simulink subsystem "Vehicle_Controller_SM_v4"  (R2023b)
settings: Solver=VariableStepAuto  StartTime=0.0  StopTime=10.0  RelTol=1e-3
undefined symbols (not defined in the file): chassis, powertrain, sensor, sim, suspension, tvs
libraries: lib_newData_range_check x4, dspstat3 x1, simulink x1
settings Model: Creator=Inver  LastModifiedBy=bowen
settings OptimizationCC: ReuseModelBlockBuffer=off

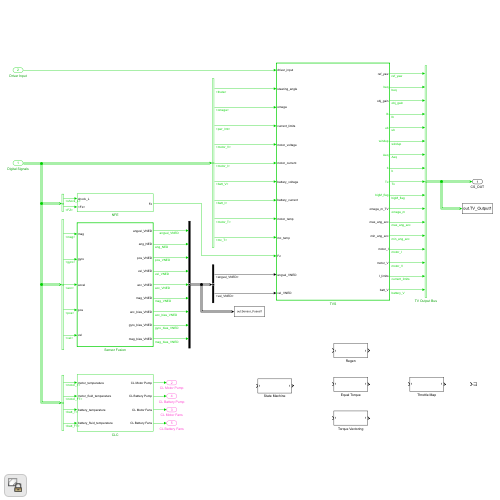
[thumbnail: Simulink's stored preview of the top-level diagram]
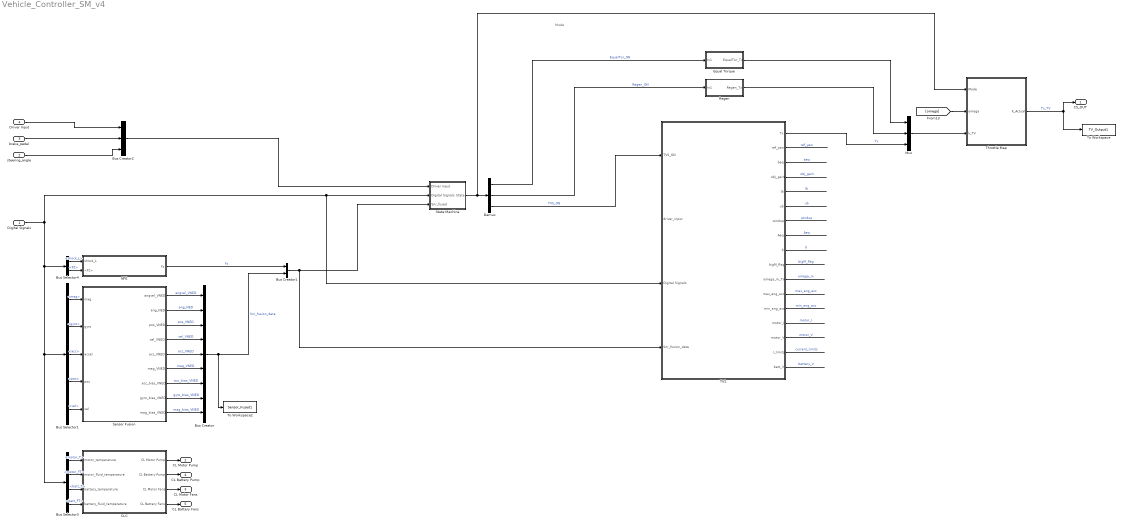
== system Vehicle_Controller_SM_v4 ==
  note: Mode
  Digital Signals : Inport
  steering_angle : Inport  Port=2
  brake_pedal : Inport  Port=3
  Driver Input : Inport  Port=4
  Bus Creator : BusCreator  Inputs=9
  Bus Creator1 : BusCreator  Inputs=2
  Bus Creator2 : BusCreator  Inputs=3
  Bus Selector1 : BusSelector  OutputSignals=Navigation Sensors.mag,Navigation Sensors.gyro,Navigation Sensors.acc,Navigation Sensors.pos,Navigation Sensors.vel
  Bus Selector3 : BusSelector  OutputSignals=Cooling Sensors.motor_T,Cooling Sensors.motor_FT,Cooling Sensors.batt_T,Cooling Sensors.batt_FT
  Bus Selector4 : BusSelector  OutputSignals=Corner Dynamics Sensors.shock_L,Corner Dynamics Sensors.FZ
  CLC : Subsystem
  Demux : Demux  Outputs=3
  Equal Torque : Subsystem
  Mux : Mux  Inputs=3
  NFE : Subsystem
  Regen : Subsystem
  Sensor Fusion : Subsystem  TreatAsAtomicUnit=on  SystemSampleTime=sim.timing.duplicate
  State Machine : Subsystem
  TVS : Subsystem  TreatAsAtomicUnit=on  SystemSampleTime=sim.timing.duplicate
  Throttle Map : Subsystem
  To Workspace : ToWorkspace  VariableName=TV_Output1  SaveFormat=Timeseries  SampleTime=-1
  To Workspace2 : ToWorkspace  VariableName=Sensor_Fused1  SaveFormat=Timeseries  SampleTime=-1
  CS_OUT : Outport
  CL Motor Pump : Outport  Port=2
  CL Motor Fans : Outport  Port=3
  CL Battery Pump : Outport  Port=4
  CL Battery Fans : Outport  Port=5
  wires:
  Sensor Fusion/4(vel_VNED) -> Bus Creator/4  "vel_VNED"
  Sensor Fusion/9(mag_bias_VNED) -> Bus Creator/9  "mag_bias_VNED"
  Bus Selector3/1 -> CLC/1(motor_temperature)  "<motor_T>"
  Bus Selector1/1 -> Sensor Fusion/1(mag)  "<mag>"
  Bus Selector3/4 -> CLC/4(battery_fluid_temperature)  "<batt_FT>"
  TVS/2(ref_yaw) -> ?  "ref_yaw"
  NFE/1(Fz) -> Bus Creator1/1  "Fz"
  Bus Selector1/2 -> Sensor Fusion/2(gyro)  "<gyro>"
  TVS/17(batt_V) -> ?  "battery_V"
  Bus Selector4/1 -> NFE/1(shock_L)  "<shock_L>"
  TVS/4(obj_gain) -> ?  "obj_gain"
  TVS/9(b) -> ?  "b"
  TVS/1(Tx) -> Mux/3  "Tx"
  Sensor Fusion/5(acc_VNED) -> Bus Creator/5  "acc_VNED"
  Bus Selector1/5 -> Sensor Fusion/5(vel)  "<vel>"
  Sensor Fusion/1(angvel_VNED) -> Bus Creator/1  "angvel_VNED"
  TVS/5(lb) -> ?  "lb"
  TVS/12(max_ang_acc) -> ?  "max_ang_acc"
  Sensor Fusion/6(mag_VNED) -> Bus Creator/6  "mag_VNED"
  CLC/1(CL Motor Pump) -> CL Motor Pump/1
  Bus Selector4/2 -> NFE/2(<Fz>)  "<FZ>"
  Bus Selector1/4 -> Sensor Fusion/4(pos)  "<pos>"
  TVS/3(beq) -> ?  "beq"
  Bus Selector3/3 -> CLC/3(battery_temperature)  "<batt_T>"
  TVS/14(motor_I) -> ?  "motor_I"
  TVS/8(Aeq) -> ?  "Aeq"
  TVS/13(min_ang_acc) -> ?  "min_ang_acc"
  Sensor Fusion/7(acc_bias_VNED) -> Bus Creator/7  "acc_bias_VNED"
  Sensor Fusion/8(gyro_bias_VNED) -> Bus Creator/8  "gyro_bias_VNED"
  TVS/7(windup) -> ?  "windup"
  CLC/4(CL Battery Fans) -> CL Battery Fans/1
  TVS/6(ub) -> ?  "ub"
  Sensor Fusion/2(ang_NED) -> Bus Creator/2  "ang_NED"
  Bus Selector1/3 -> Sensor Fusion/3(accel)  "<acc>"
  TVS/10(bigM_flag) -> ?  "bigM_flag"
  TVS/15(motor_V) -> ?  "motor_V"
  TVS/11(omega_m_TV) -> ?  "omega_m"
  TVS/16(I_limits) -> ?  "current_limits"
  Bus Selector3/2 -> CLC/2(motor_fluid_temperature)  "<motor_FT>"
  Sensor Fusion/3(pos_VNED) -> Bus Creator/3  "pos_VNED"
  Bus Creator/1 -> To Workspace2/1, Bus Creator1/2  "Snr_fusion_data"
  CLC/3(CL Motor Fans) -> CL Motor Fans/1
  CLC/2(CL Battery Pump) -> CL Battery Pump/1
  Bus Creator1/1 -> State Machine/3(Snr_fused), TVS/4(Snr_fusion_data)
  [omega] -> Throttle Map/2(omega)
  Throttle Map/1(K_Actual) -> CS_OUT/1, To Workspace/1  "Tx_TV"
  Digital Signals/1 -> State Machine/2(Digital Signals), TVS/3(Digital Signals), Bus Selector3/1, Bus Selector1/1, Bus Selector4/1
  State Machine/1(State) -> Demux/1, Throttle Map/1(Mode)
  Demux/1 -> Equal Torque/1(In1)  "EqualTor_ON"
  Demux/2 -> Regen/1(In1)  "Regen_ON"
  Demux/3 -> TVS/1(TVS_ON)  "TVS_ON"
  Equal Torque/1(EqualTor_Tx) -> Mux/1
  Mux/1 -> Throttle Map/3(k_TV)
  Regen/1(Regen_Tx) -> Mux/2
  Driver Input/1 -> Bus Creator2/1
  steering_angle/1 -> Bus Creator2/3
  brake_pedal/1 -> Bus Creator2/2
  Bus Creator2/1 -> State Machine/1(Driver Input)

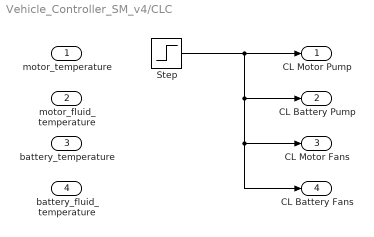
== system Vehicle_Controller_SM_v4/CLC ==
  motor_temperature : Inport
  motor_fluid_temperature : Inport  Port=2
  battery_temperature : Inport  Port=3
  battery_fluid_temperature : Inport  Port=4
  Step : Step  After=0  SampleTime=0
  CL Motor Pump : Outport
  CL Battery Pump : Outport  Port=2
  CL Motor Fans : Outport  Port=3
  CL Battery Fans : Outport  Port=4
  wires:
  Step/1 -> CL Motor Fans/1, CL Battery Fans/1, CL Battery Pump/1, CL Motor Pump/1

== system Vehicle_Controller_SM_v4/Equal Torque ==
  In1 : Inport
  Constant{,1..3} (4 alike) : Constant  OutDataTypeStr=double
  Tx_RAW_demux : Mux
  EqualTor_Tx : Outport
  wires:
  Constant1/1 -> Tx_RAW_demux/2  "TFR"
  Constant2/1 -> Tx_RAW_demux/3  "TRL"
  Tx_RAW_demux/1 -> EqualTor_Tx/1  "Tx_RAW_TV"
  Constant/1 -> Tx_RAW_demux/1  "TFL"
  Constant3/1 -> Tx_RAW_demux/4  "TRR"

== system Vehicle_Controller_SM_v4/NFE ==
  shock_L : Inport
  <Fz> : Inport  Port=2
  Saturation17 : Saturate  UpperLimit=1200  LowerLimit=200
  Terminator : Terminator
  Fz : Outport
  wires:
  shock_L/1 -> Terminator/1
  <Fz>/1 -> Saturation17/1
  Saturation17/1 -> Fz/1  "FZ"

== system Vehicle_Controller_SM_v4/Regen ==
  In1 : Inport
  Constant{,1..3} (4 alike) : Constant  Value=0
  Tx_RAW_demux : Mux
  Regen_Tx : Outport
  wires:
  Tx_RAW_demux/1 -> Regen_Tx/1  "Tx_RAW_TV"
  Constant3/1 -> Tx_RAW_demux/4  "TRR"
  Constant1/1 -> Tx_RAW_demux/2  "TFR"
  Constant/1 -> Tx_RAW_demux/1  "TFL"
  Constant2/1 -> Tx_RAW_demux/3  "TRL"

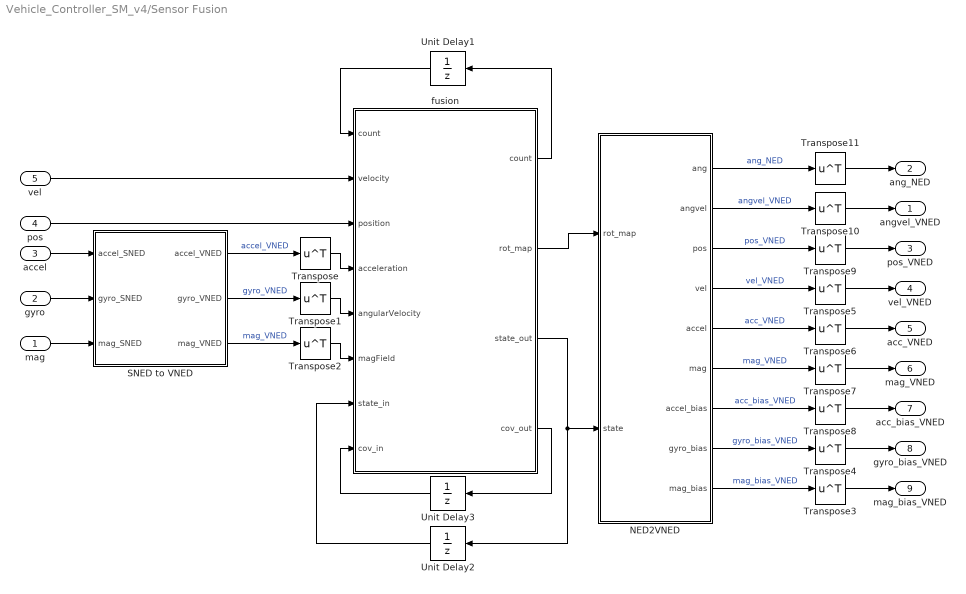
== system Vehicle_Controller_SM_v4/Sensor Fusion ==
  mag : Inport
  gyro : Inport  Port=2
  accel : Inport  Port=3
  pos : Inport  Port=4
  vel : Inport  Port=5
  NED2VNED : MATLAB Function  TreatAsAtomicUnit=on
  SNED to VNED : MATLAB Function  TreatAsAtomicUnit=on
  Transpose{,1..11} (12 alike) : Math  Operator=transpose
  Unit Delay1 : UnitDelay  InitialCondition=sim.IC.gps_counter_IC  SampleTime=-1  HasFrameUpgradeWarning=on
  Unit Delay2 : UnitDelay  InitialCondition=sim.IC.state_IC  SampleTime=-1  HasFrameUpgradeWarning=on
  Unit Delay3 : UnitDelay  InitialCondition=sim.IC.covarience_matrix_IC  SampleTime=-1  HasFrameUpgradeWarning=on
  fusion : MATLAB Function  TreatAsAtomicUnit=on
  angvel_VNED : Outport
  ang_NED : Outport  Port=2
  pos_VNED : Outport  Port=3
  vel_VNED : Outport  Port=4
  acc_VNED : Outport  Port=5
  mag_VNED : Outport  Port=6
  acc_bias_VNED : Outport  Port=7
  gyro_bias_VNED : Outport  Port=8
  mag_bias_VNED : Outport  Port=9
  wires:
  NED2VNED/7(accel_bias) -> Transpose8/1  "acc_bias_VNED"
  NED2VNED/3(pos) -> Transpose9/1  "pos_VNED"
  NED2VNED/4(vel) -> Transpose5/1  "vel_VNED"
  NED2VNED/2(angvel) -> Transpose10/1  "angvel_VNED"
  NED2VNED/1(ang) -> Transpose11/1  "ang_NED"
  fusion/2(rot_map) -> NED2VNED/1(rot_map)
  Transpose/1 -> fusion/4(acceleration)
  Unit Delay3/1 -> fusion/8(cov_in)
  NED2VNED/8(gyro_bias) -> Transpose4/1  "gyro_bias_VNED"
  Transpose1/1 -> fusion/5(angularVelocity)
  fusion/4(cov_out) -> Unit Delay3/1
  fusion/3(state_out) -> Unit Delay2/1, NED2VNED/2(state)
  SNED to VNED/2(gyro_VNED) -> Transpose1/1  "gyro_VNED"
  SNED to VNED/1(accel_VNED) -> Transpose/1  "accel_VNED"
  NED2VNED/5(accel) -> Transpose6/1  "acc_VNED"
  SNED to VNED/3(mag_VNED) -> Transpose2/1  "mag_VNED"
  Unit Delay2/1 -> fusion/7(state_in)
  Transpose2/1 -> fusion/6(magField)
  NED2VNED/9(mag_bias) -> Transpose3/1  "mag_bias_VNED"
  NED2VNED/6(mag) -> Transpose7/1  "mag_VNED"
  accel/1 -> SNED to VNED/1(accel_SNED)
  gyro/1 -> SNED to VNED/2(gyro_SNED)
  mag/1 -> SNED to VNED/3(mag_SNED)
  pos/1 -> fusion/3(position)
  vel/1 -> fusion/2(velocity)
  Transpose3/1 -> mag_bias_VNED/1
  Transpose4/1 -> gyro_bias_VNED/1
  Transpose8/1 -> acc_bias_VNED/1
  Transpose7/1 -> mag_VNED/1
  Transpose6/1 -> acc_VNED/1
  Transpose5/1 -> vel_VNED/1
  Transpose9/1 -> pos_VNED/1
  Transpose10/1 -> angvel_VNED/1
  Transpose11/1 -> ang_NED/1
  fusion/1(count) -> Unit Delay1/1
  Unit Delay1/1 -> fusion/1("count ")

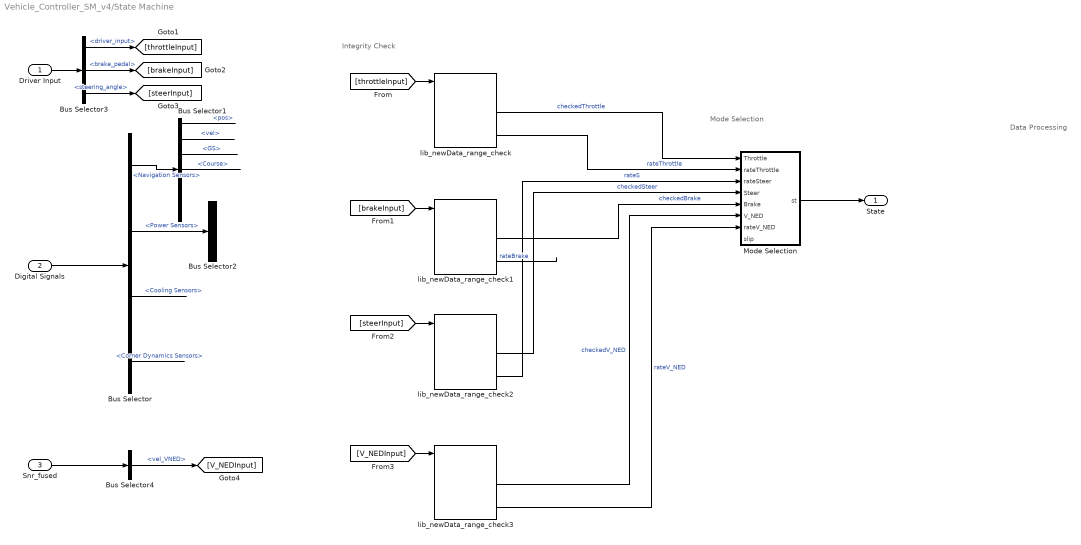
== system Vehicle_Controller_SM_v4/State Machine ==
  note: Mode Selection
  note: Data Processing
  note: Integrity Check
  Driver Input : Inport
  Digital Signals : Inport  Port=2
  Snr_fused : Inport  Port=3
  Bus Selector : BusSelector  OutputSignals=Navigation Sensors,Power Sensors,Cooling Sensors,Corner Dynamics Sensors
  Bus Selector1 : BusSelector  OutputSignals=pos,vel,GS,Course,acc,gyro,mag
  Bus Selector2 : BusSelector  OutputSignals=batt_V,batt_I,motor_V,motor_I,pwr_lmt
  Bus Selector3 : BusSelector  OutputSignals=driver_input,brake_pedal,steering_angle
  Bus Selector4 : BusSelector  OutputSignals=Snr_fusion_data.vel_VNED
  Mode Selection : Stateflow chart  TreatAsAtomicUnit=on
      settings: PortSchema="{\"entries\":[{\"content\":{\"sides\":[{\"content\":{\"connectorIds\":[\"In2\",\"In1\",\"In3\",\"In4\",\"In5\",\"In6\",\"In7\",\"In8\"]},\"type\":\"ConnectorPlacement.EquallySpacedRectSide\",\"uuid\":\"6558decb-560a-4e99-886a-7df098711fc6\"},{\"content\":{\"connectorIds\":[\"Out1\"],\"side\":\"RIGHT\"},\"type\":\"ConnectorPlacement.EquallySpacedRectSide\",\"uuid\":\"f716a093-64f4-43ea-8871-c60e18977aa6\"},{\"content\":{\"side\":\"TOP\"},\"type\":\"ConnectorPlacement.EquallySpacedRectSide\",\"uuid\":\"8a2fdf23-ff95-496c-b229-9a5a43c5cbff\"}]},\"type\":\"ConnectorPlacement.EquallySpacedConnector\",\"uuid\":\"3c12f053-2241-41ba-99fa-529980201ae5\"}],\"packageUris\":[\"http://schema.mathworks.com/mf0/Connector/R2020b\"],\"version\":\"1.0\"}"
  lib_newData_range_check{,1..3} (4 alike) : lib_newData_range_check/lib_newData_range_check  SystemSampleTime=-1  VariantActivationTime=update diagram  AllowFlexibleInterface=on  Latency=0  AutoFrameSizeCalculation=off
  State : Outport  PortDimensions=[3 1]
  wires:
  [V_NEDInput] -> lib_newData_range_check3/1
  lib_newData_range_check3/2 -> Mode Selection/6(V_NED)  "checkedV_NED"
  lib_newData_range_check3/3 -> Mode Selection/7(rateV_NED)  "rateV_NED"
  [steerInput] -> lib_newData_range_check2/1
  [brakeInput] -> lib_newData_range_check1/1
  lib_newData_range_check2/2 -> Mode Selection/4(Steer)  "checkedSteer"
  lib_newData_range_check2/3 -> Mode Selection/3(rateSteer)  "rateS"
  lib_newData_range_check1/2 -> Mode Selection/5(Brake)  "checkedBrake"
  lib_newData_range_check1/3 -> ?  "rateBrake"
  [throttleInput] -> lib_newData_range_check/1
  lib_newData_range_check/3 -> Mode Selection/1(rateThrottle)  "rateThrottle"
  lib_newData_range_check/2 -> Mode Selection/2(Throttle)  "checkedThrottle"
  Bus Selector3/3 -> [steerInput]  "<steering_angle>"
  Bus Selector3/2 -> [brakeInput]  "<brake_pedal>"
  Bus Selector3/1 -> [throttleInput]  "<driver_input>"
  Bus Selector4/1 -> [V_NEDInput]  "<vel_VNED>"
  Snr_fused/1 -> Bus Selector4/1
  Driver Input/1 -> Bus Selector3/1
  Mode Selection/1(st) -> State/1
  Bus Selector1/4 -> ?  "<Course>"
  Bus Selector1/3 -> ?  "<GS>"
  Bus Selector1/2 -> ?  "<vel>"
  Bus Selector1/1 -> ?  "<pos>"
  Bus Selector/4 -> ?  "<Corner Dynamics Sensors>"
  Bus Selector/3 -> ?  "<Cooling Sensors>"
  Bus Selector/2 -> Bus Selector2/1  "<Power Sensors>"
  Bus Selector/1 -> Bus Selector1/1  "<Navigation Sensors>"
  Digital Signals/1 -> Bus Selector/1

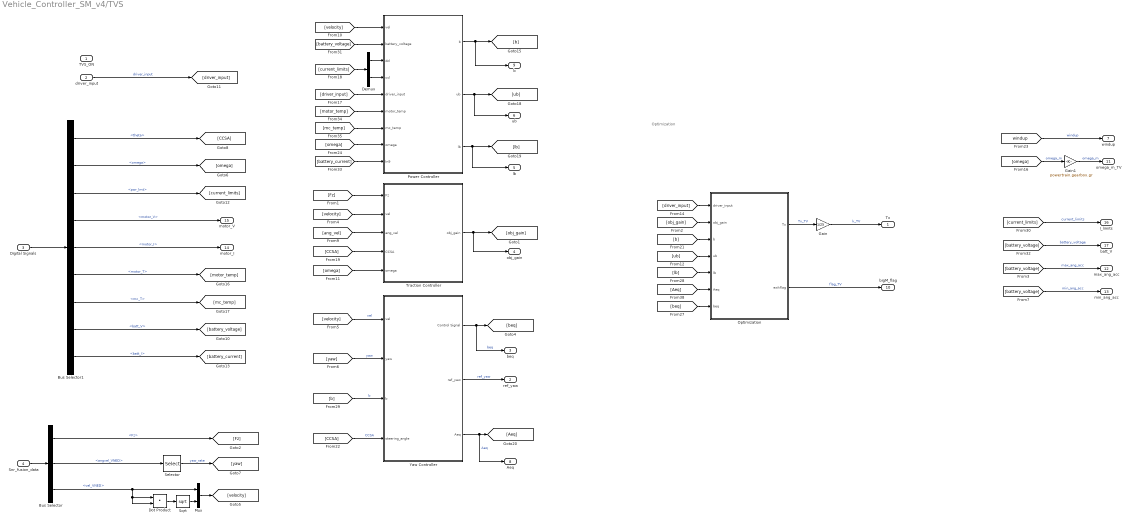
== system Vehicle_Controller_SM_v4/TVS ==
  note: Optimization
  TVS_ON : Inport
  driver_input : Inport  Port=2  OutMin=-1  OutMax=1  OutDataTypeStr=double  PortDimensions=1  LockScale=on
  Digital Signals : Inport  Port=3
  Snr_fusion_data : Inport  Port=4
  Bus Selector : BusSelector  OutputSignals=Fz,Snr_fusion_data.angvel_VNED,Snr_fusion_data.vel_VNED
  Bus Selector1 : BusSelector  OutputSignals=Corner Dynamics Sensors.theta,Corner Dynamics Sensors.omega,Power Sensors.pwr_lmt,Power Sensors.motor_V,Power Sensors.motor_I,Cooling Sensors.motor_T,Cooling Sensors.mc_T,Power Sensors.batt_V,Power Sensors.batt_I
  Demux : Demux  Outputs=2
  Dot Product : DotProduct  OutDataTypeStr=Inherit: Inherit via internal rule
  Gain : Gain  Gain=1/25
  Gain1 : Gain  Gain=powertrain.gearbox.gr  ParamDataTypeStr=double  OutDataTypeStr=Inherit: Inherit via back propagation
  Mux : Mux  Inputs=2
  Optimization : Subsystem
  Power Controller : Subsystem
  Selector : Selector  InputPortWidth=3  IndexOptions=Index vector (dialog)  Indices=3  OutputSizes=1
  Sqrt : Sqrt
  Traction Controller : Subsystem
  Yaw Controller : Subsystem
  Tx : Outport  OutDataTypeStr=double  PortDimensions=[1 4]
  ref_yaw : Outport  Port=2
  beq : Outport  Port=3  OutMin=-10  OutMax=10  OutDataTypeStr=double  LockScale=on
  obj_gain : Outport  Port=4
  lb : Outport  Port=5  OutMin=-25  OutMax=25  OutDataTypeStr=double  LockScale=on
  ub : Outport  Port=6  OutMin=-25  OutMax=25  OutDataTypeStr=double  LockScale=on
  windup : Outport  Port=7
  Aeq : Outport  Port=8  OutMin=-1.9  OutMax=1.9  OutDataTypeStr=double  LockScale=on
  b : Outport  Port=9  OutMin=-80000  OutMax=80000  OutDataTypeStr=double  LockScale=on
  bigM_flag : Outport  Port=10  PortDimensions=1
  omega_m_TV : Outport  Port=11
  max_ang_acc : Outport  Port=12
  min_ang_acc : Outport  Port=13
  motor_I : Outport  Port=14
  motor_V : Outport  Port=15
  I_limits : Outport  Port=16
  batt_V : Outport  Port=17
  wires:
  Bus Selector1/7 -> [mc_temp]  "<mc_T>"
  Bus Selector1/8 -> [battery_voltage]  "<batt_V>"
  Bus Selector1/9 -> [battery_current]  "<batt_I>"
  Bus Selector1/6 -> [motor_temp]  "<motor_T>"
  Bus Selector1/5 -> motor_I/1  "<motor_I>"
  Bus Selector1/4 -> motor_V/1  "<motor_V>"
  Bus Selector1/3 -> [current_limits]  "<pwr_lmt>"
  Bus Selector1/2 -> [omega]  "<omega>"
  Bus Selector1/1 -> [CCSA]  "<theta>"
  Digital Signals/1 -> Bus Selector1/1
  Bus Selector/3 -> Mux/1, Dot Product/1, Dot Product/2  "<vel_VNED>"
  Bus Selector/1 -> [Fz]  "<Fz>"
  Bus Selector/2 -> Selector/1  "<angvel_VNED>"
  Snr_fusion_data/1 -> Bus Selector/1
  [velocity] -> Traction Controller/2(vel)
  Optimization/2(exitflag) -> bigM_flag/1  "flag_TV"
  [omega] -> Gain1/1  "omega_m"
  [velocity] -> Yaw Controller/1(vel)  "vel"
  [ang_vel] -> Traction Controller/3(ang_vel)
  Power Controller/1(b) -> [b], b/1
  Traction Controller/1(obj_gain) -> [obj_gain], obj_gain/1
  Power Controller/2(ub) -> ub/1, [ub]
  [omega] -> Traction Controller/5(omega)
  [driver_input] -> Optimization/1(driver_input)
  Yaw Controller/1(Control Signal) -> [beq], beq/1  "beq"
  [yaw] -> Yaw Controller/2(yaw)  "yaw"
  [Fz] -> Traction Controller/1(Fz)
  [windup] -> windup/1  "windup"
  Yaw Controller/3(Aeq) -> [Aeq], Aeq/1  "Aeq"
  driver_input/1 -> [driver_input]  "driver_input"
  [beq] -> Optimization/7(beq)
  Power Controller/3(lb) -> lb/1, [lb]
  [obj_gain] -> Optimization/2(obj_gain)
  Yaw Controller/2(ref_yaw) -> ref_yaw/1  "ref_yaw"
  [current_limits] -> I_limits/1  "current_limits"
  [battery_voltage] -> batt_V/1  "battery_voltage"
  Selector/1 -> [yaw]  "yaw_rate"
  Dot Product/1 -> Sqrt/1
  Mux/1 -> [velocity]
  Sqrt/1 -> Mux/2
  Gain1/1 -> omega_m_TV/1  "omega_m"
  [CCSA] -> Traction Controller/4(CCSA)
  [velocity] -> Power Controller/1(vel)
  [battery_voltage] -> Power Controller/2(battery_voltage)
  [battery_current] -> Power Controller/9(In9)
  [driver_input] -> Power Controller/5(driver_input)
  [motor_temp] -> Power Controller/6(motor_temp)
  [mc_temp] -> Power Controller/7(mc_temp)
  [current_limits] -> Demux/1
  Demux/2 -> Power Controller/4(ccl)
  Demux/1 -> Power Controller/3(dcl)
  [CCSA] -> Yaw Controller/4(steering_angle)  "CCSA"
  [ub] -> Optimization/4(ub)
  [lb] -> Optimization/5(lb)
  [b] -> Optimization/3(b)
  [b] -> Yaw Controller/3(b)  "b"
  [Aeq] -> Optimization/6(Aeq)
  [omega] -> Power Controller/8(omega)
  [battery_voltage] -> max_ang_acc/1  "max_ang_acc"
  [battery_voltage] -> min_ang_acc/1  "min_ang_acc"
  Gain/1 -> Tx/1  "k_TV"
  Optimization/1(Tx) -> Gain/1  "Tx_TV"

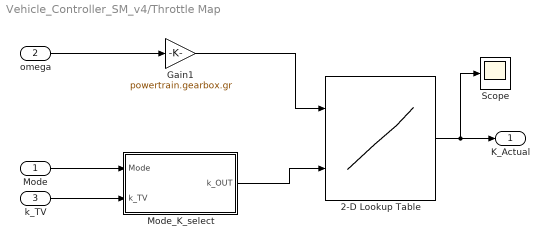
== system Vehicle_Controller_SM_v4/Throttle Map ==
  Mode : Inport
  omega : Inport  Port=2
  k_TV : Inport  Port=3
  2-D Lookup Table : Lookup_n-D  LookupTableObject=''  BreakpointsForDimension1=tvs.torque_control.omega_bp  BreakpointsForDimension2=tvs.torque_control.k_linear_bp  BreakpointsForDimension1FirstPoint=10  BreakpointsForDimension2FirstPoint=10  BreakpointsForDimension1Spacing=12  BreakpointsForDimension2Spacing=12  Table=tvs.torque_control.k_actual  ExtrapMethod=Clip  DiagnosticForOutOfRangeInput=Error  InternalRulePriority=Speed  RndMeth=Simplest
      settings: InputPortMap=u0,u1
  Gain1 : Gain  Gain=powertrain.gearbox.gr
  Mode_K_select : MATLAB Function  TreatAsAtomicUnit=on
  Scope : Scope
  K_Actual : Outport
  wires:
  2-D Lookup Table/1 -> K_Actual/1, Scope/1
  Mode_K_select/1(k_OUT) -> 2-D Lookup Table/2
  Mode/1 -> Mode_K_select/1(Mode)
  k_TV/1 -> Mode_K_select/2(k_TV)
  omega/1 -> Gain1/1
  Gain1/1 -> 2-D Lookup Table/1

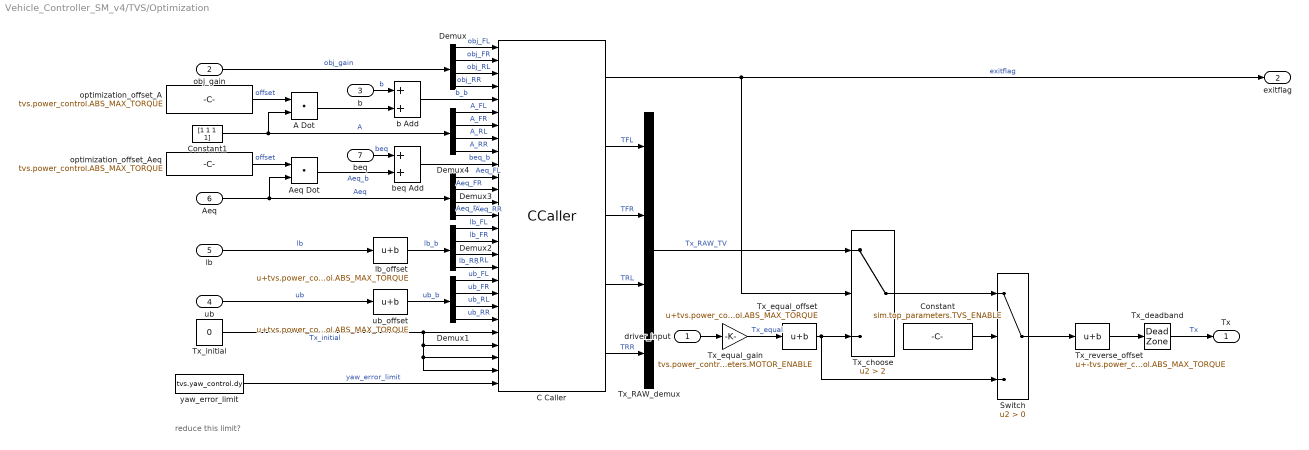
== system Vehicle_Controller_SM_v4/TVS/Optimization ==
  note: reduce this limit?
  driver_input : Inport  OutDataTypeStr=double
  obj_gain : Inport  Port=2
  b : Inport  Port=3  OutDataTypeStr=double
  ub : Inport  Port=4  OutDataTypeStr=double
  lb : Inport  Port=5  OutDataTypeStr=double
  Aeq : Inport  Port=6  OutDataTypeStr=double
  beq : Inport  Port=7  OutDataTypeStr=double
  A Dot : DotProduct  OutDataTypeStr=double
  Aeq Dot : DotProduct  OutDataTypeStr=double
  C Caller : CCaller  FunctionName=bigM_func
  Constant : Constant  Value=sim.top_parameters.TVS_ENABLE
  Constant1 : Constant  Value=[1 1 1 1]
  Demux{,1..4} (5 alike) : Demux
  Switch : Switch  Criteria=u2 > Threshold  SaturateOnIntegerOverflow=off  InputSameDT=off
  Tx_RAW_demux : Mux
  Tx_choose : Switch  Criteria=u2 > Threshold  Threshold=2  OutDataTypeStr=double  SaturateOnIntegerOverflow=off  InputSameDT=off
  Tx_deadband : DeadZone  LowerValue=-10*tvs.power_control.dTx  UpperValue=10*tvs.power_control.dTx
  Tx_equal_gain : Gain  Gain=tvs.power_control.ABS_MAX_TORQUE.*sim.top_parameters.MOTOR_ENABLE  OutDataTypeStr=double
  Tx_equal_offset : Bias  Bias=tvs.power_control.ABS_MAX_TORQUE  SaturateOnIntegerOverflow=off
  Tx_initial : Constant  Value=0  OutDataTypeStr=double
  Tx_reverse_offset : Bias  Bias=-tvs.power_control.ABS_MAX_TORQUE  SaturateOnIntegerOverflow=off
  b Add : Sum  OutDataTypeStr=double
  beq Add : Sum  OutDataTypeStr=double
  lb_offset : Bias  Bias=tvs.power_control.ABS_MAX_TORQUE  SaturateOnIntegerOverflow=off
  optimization_offset_A : Constant  Value=tvs.power_control.ABS_MAX_TORQUE  OutDataTypeStr=double
  optimization_offset_Aeq : Constant  Value=tvs.power_control.ABS_MAX_TORQUE  OutDataTypeStr=double
  ub_offset : Bias  Bias=tvs.power_control.ABS_MAX_TORQUE  SaturateOnIntegerOverflow=off
  yaw_error_limit : Constant  Value=tvs.yaw_control.dy  OutDataTypeStr=double
  Tx : Outport
  exitflag : Outport  Port=2
  wires:
  C Caller/1 -> Tx_choose/2, exitflag/1  "exitflag"
  lb/1 -> lb_offset/1  "lb"
  ub/1 -> ub_offset/1  "ub"
  C Caller/2 -> Tx_RAW_demux/1  "TFL"
  C Caller/5 -> Tx_RAW_demux/4  "TRR"
  C Caller/4 -> Tx_RAW_demux/3  "TRL"
  C Caller/3 -> Tx_RAW_demux/2  "TFR"
  Demux/1 -> C Caller/1  "obj_FL"
  Demux/2 -> C Caller/2  "obj_FR"
  Demux/3 -> C Caller/3  "obj_RL"
  Demux/4 -> C Caller/4  "obj_RR"
  Tx_initial/1 -> C Caller/23, C Caller/24, C Caller/25, C Caller/26  "Tx_initial"
  Demux1/1 -> C Caller/19  "ub_FL"
  Demux1/2 -> C Caller/20  "ub_FR"
  Demux1/3 -> C Caller/21  "ub_RL"
  Demux1/4 -> C Caller/22  "ub_RR"
  Demux2/1 -> C Caller/15  "lb_FL"
  Demux2/2 -> C Caller/16  "lb_FR"
  Demux2/3 -> C Caller/17  "lb_RL"
  Demux2/4 -> C Caller/18  "lb_RR"
  Demux3/3 -> C Caller/13  "Aeq_RL"
  Demux3/2 -> C Caller/12  "Aeq_FR"
  Demux3/1 -> C Caller/11  "Aeq_FL"
  Demux3/4 -> C Caller/14  "Aeq_RR"
  Demux4/1 -> C Caller/6  "A_FL"
  Demux4/2 -> C Caller/7  "A_FR"
  Demux4/3 -> C Caller/8  "A_RL"
  Demux4/4 -> C Caller/9  "A_RR"
  ub_offset/1 -> Demux1/1  "ub_b"
  optimization_offset_Aeq/1 -> Aeq Dot/1  "offset"
  optimization_offset_A/1 -> A Dot/1  "offset"
  beq/1 -> beq Add/1  "beq"
  Aeq Dot/1 -> beq Add/2  "Aeq_b"
  b/1 -> b Add/1  "b"
  A Dot/1 -> b Add/2
  yaw_error_limit/1 -> C Caller/27  "yaw_error_limit"
  Tx_RAW_demux/1 -> Tx_choose/1  "Tx_RAW_TV"
  Constant1/1 -> Demux4/1, A Dot/2  "A"
  b Add/1 -> C Caller/5  "b_b"
  obj_gain/1 -> Demux/1  "obj_gain"
  lb_offset/1 -> Demux2/1  "lb_b"
  Aeq/1 -> Demux3/1, Aeq Dot/2  "Aeq"
  beq Add/1 -> C Caller/10  "beq_b"
  Tx_deadband/1 -> Tx/1  "Tx"
  Tx_reverse_offset/1 -> Tx_deadband/1
  driver_input/1 -> Tx_equal_gain/1
  Tx_choose/1 -> Switch/1
  Tx_equal_gain/1 -> Tx_equal_offset/1  "Tx_equal"
  Tx_equal_offset/1 -> Switch/3, Tx_choose/3
  Switch/1 -> Tx_reverse_offset/1
  Constant/1 -> Switch/2

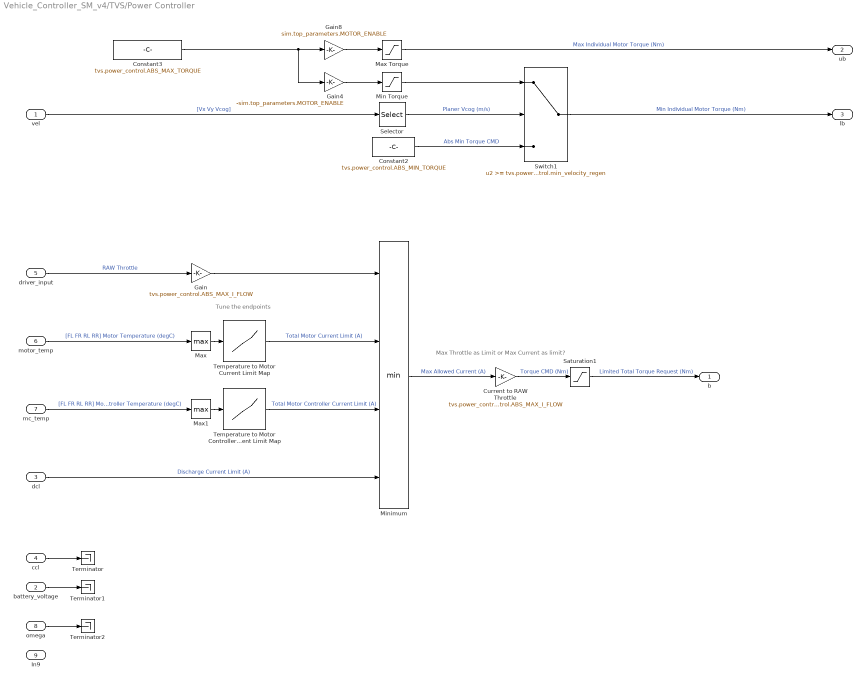
== system Vehicle_Controller_SM_v4/TVS/Power Controller ==
  note: Max Throttle as Limit or Max Current as limit?
  note: Tune the endpoints
  vel : Inport  OutDataTypeStr=double
  battery_voltage : Inport  Port=2
  dcl : Inport  Port=3  OutDataTypeStr=double  LockScale=on
  ccl : Inport  Port=4  OutDataTypeStr=double  LockScale=on
  driver_input : Inport  Port=5  OutDataTypeStr=double  LockScale=on
  motor_temp : Inport  Port=6
  mc_temp : Inport  Port=7
  omega : Inport  Port=8
  In9 : Inport  Port=9
  Constant2 : Constant  Value=tvs.power_control.ABS_MIN_TORQUE  OutDataTypeStr=double
  Constant3 : Constant  Value=tvs.power_control.ABS_MAX_TORQUE
  Current to RAW Throttle : Gain  Gain=tvs.power_control.ABS_MAX_TRQ_CMD/tvs.power_control.ABS_MAX_I_FLOW
  Gain : Gain  Gain=tvs.power_control.ABS_MAX_I_FLOW
  Gain4 : Gain  Gain=-sim.top_parameters.MOTOR_ENABLE  ParamDataTypeStr=double  OutDataTypeStr=Inherit: Inherit via back propagation
  Gain8 : Gain  Gain=sim.top_parameters.MOTOR_ENABLE  ParamDataTypeStr=double  OutDataTypeStr=Inherit: Inherit via back propagation
  Max : MinMax  Function=max
  Max Torque : Saturate  UpperLimit=tvs.power_control.ABS_MAX_TORQUE  LowerLimit=2.*tvs.power_control.dTx  OutDataTypeStr=Inherit: Inherit via back propagation
  Max1 : MinMax  Function=max
  Min Torque : Saturate  UpperLimit=tvs.power_control.dTx  LowerLimit=tvs.power_control.ABS_MIN_TORQUE  OutDataTypeStr=Inherit: Inherit via back propagation
  Minimum : MinMax  Inputs=4
  Saturation1 : Saturate  UpperLimit=tvs.power_control.ABS_MAX_TRQ_CMD  LowerLimit=tvs.power_control.ABS_MIN_TRQ_CMD
  Selector : Selector  InputPortWidth=4  IndexOptions=Index vector (dialog)  Indices=4  OutputSizes=1
  Switch1 : Switch  Threshold=tvs.power_control.min_velocity_regen  OutDataTypeStr=Inherit: Inherit via back propagation  SaturateOnIntegerOverflow=off  InputSameDT=off
  Temperature to Motor Controller Current Limit Map : Lookup_n-D  NumberOfTableDimensions=1  BreakpointsForDimension1=tvs.power_control.motor_controller_t_bp  IndexSearchMethod=Evenly spaced points  Table=tvs.power_control.motor_controller_I_table  ExtrapMethod=Clip  UseLastTableValue=on  InternalRulePriority=Speed  RndMeth=Simplest
  Temperature to Motor Current Limit Map : Lookup_n-D  NumberOfTableDimensions=1  BreakpointsForDimension1=tvs.power_control.motor_t_bp  IndexSearchMethod=Evenly spaced points  Table=tvs.power_control.motor_I_table  ExtrapMethod=Clip  UseLastTableValue=on  InternalRulePriority=Speed  RndMeth=Simplest
  Terminator : Terminator
  Terminator1 : Terminator
  Terminator2 : Terminator
  b : Outport  OutDataTypeStr=double  LockScale=on
  ub : Outport  Port=2  OutDataTypeStr=double  LockScale=on
  lb : Outport  Port=3  OutDataTypeStr=double  LockScale=on
  wires:
  Max1/1 -> Temperature to Motor Controller Current Limit Map/1
  Temperature to Motor Current Limit Map/1 -> Minimum/2  "Total Motor Current Limit (A)"
  battery_voltage/1 -> Terminator1/1
  Gain8/1 -> Max Torque/1
  Constant3/1 -> Gain4/1, Gain8/1
  Max/1 -> Temperature to Motor Current Limit Map/1
  Gain4/1 -> Min Torque/1
  Constant2/1 -> Switch1/3  "Abs Min Torque CMD"
  Selector/1 -> Switch1/2  "Planer Vcog (m/s)"
  motor_temp/1 -> Max/1  "[FL FR RL RR] Motor Temperature (degC)"
  ccl/1 -> Terminator/1
  driver_input/1 -> Gain/1  "RAW Throttle"
  Max Torque/1 -> ub/1  "Max Individual Motor Torque (Nm)"
  Gain/1 -> Minimum/1
  mc_temp/1 -> Max1/1  "[FL FR RL RR] Motor Controller Temperature (degC)"
  dcl/1 -> Minimum/4  "Discharge Current Limit (A)"
  vel/1 -> Selector/1  "[Vx Vy Vcog]"
  Temperature to Motor Controller Current Limit Map/1 -> Minimum/3  "Total Motor Controller Current Limit (A)"
  Min Torque/1 -> Switch1/1
  Switch1/1 -> lb/1  "Min Individual Motor Torque (Nm)"
  Minimum/1 -> Current to RAW Throttle/1  "Max Allowed Current (A)"
  omega/1 -> Terminator2/1
  Saturation1/1 -> b/1  "Limited Total Torque Request (Nm)"
  Current to RAW Throttle/1 -> Saturation1/1  "Torque CMD (Nm)"

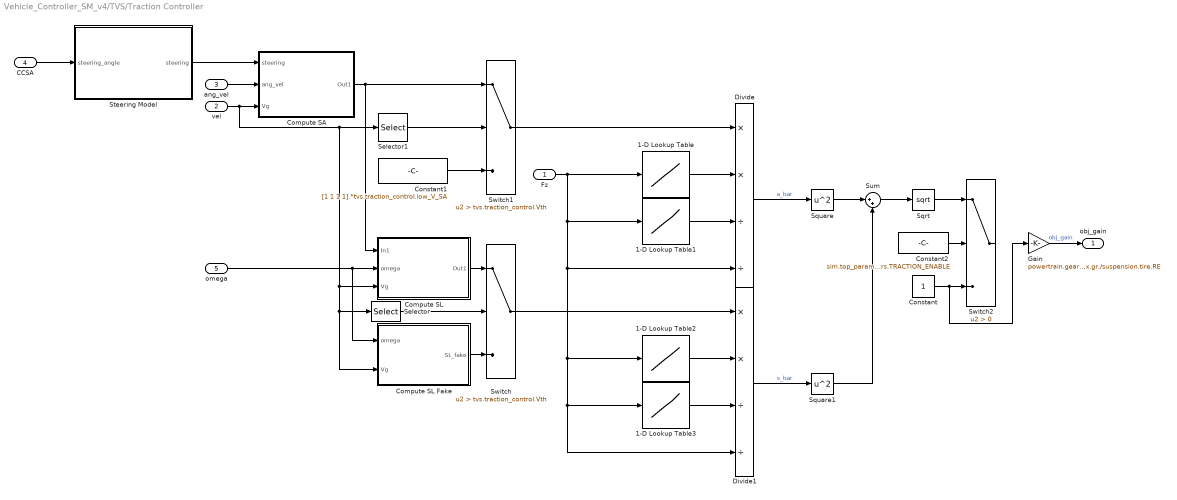
== system Vehicle_Controller_SM_v4/TVS/Traction Controller ==
  Fz : Inport  OutDataTypeStr=double  LockScale=on
  vel : Inport  Port=2  OutDataTypeStr=double  LockScale=on
  ang_vel : Inport  Port=3  OutDataTypeStr=double  LockScale=on
  CCSA : Inport  Port=4
  omega : Inport  Port=5
  1-D Lookup Table : Lookup_n-D  NumberOfTableDimensions=1  BreakpointsForDimension1=suspension.tire.Fz_sweep  Table=suspension.tire.cy_sweep  InternalRulePriority=Speed  RndMeth=Simplest
  1-D Lookup Table1 : Lookup_n-D  NumberOfTableDimensions=1  BreakpointsForDimension1=suspension.tire.Fz_sweep  Table=suspension.tire.my_sweep  InternalRulePriority=Speed  RndMeth=Simplest
  1-D Lookup Table2 : Lookup_n-D  NumberOfTableDimensions=1  BreakpointsForDimension1=suspension.tire.Fz_sweep  Table=suspension.tire.kx_sweep  InternalRulePriority=Speed  RndMeth=Simplest
  1-D Lookup Table3 : Lookup_n-D  NumberOfTableDimensions=1  BreakpointsForDimension1=suspension.tire.Fz_sweep  Table=suspension.tire.mx_sweep  InternalRulePriority=Speed  RndMeth=Simplest
  Compute SA : Subsystem
  Compute SL : Subsystem
  Compute SL Fake : Subsystem
  Constant : Constant
  Constant1 : Constant  Value=[1 1 1 1].*tvs.traction_control.low_V_SA
  Constant2 : Constant  Value=sim.top_parameters.TRACTION_ENABLE
  Divide : Product  Inputs=**//
  Divide1 : Product  Inputs=**//
  Gain : Gain  Gain=powertrain.gearbox.gr./suspension.tire.RE
  Selector : Selector  InputPortWidth=4  IndexOptions=Index vector (dialog)  Indices=4  OutputSizes=1
  Selector1 : Selector  InputPortWidth=4  IndexOptions=Index vector (dialog)  Indices=4  OutputSizes=1
  Sqrt : Sqrt
  Square : Math  Operator=square
  Square1 : Math  Operator=square
  Steering Model : Subsystem
  Sum : Sum  Inputs=|++
  Switch : Switch  Criteria=u2 > Threshold  Threshold=tvs.traction_control.Vth  SaturateOnIntegerOverflow=off  InputSameDT=off
  Switch1 : Switch  Criteria=u2 > Threshold  Threshold=tvs.traction_control.Vth  SaturateOnIntegerOverflow=off  InputSameDT=off
  Switch2 : Switch  Criteria=u2 > Threshold  SaturateOnIntegerOverflow=off  InputSameDT=off
  obj_gain : Outport
  wires:
  Gain/1 -> obj_gain/1  "obj_gain"
  Constant/1 -> Gain/1, Switch2/3
  Sum/1 -> Sqrt/1
  Divide/1 -> Square/1  "a_bar"
  1-D Lookup Table/1 -> Divide/2
  1-D Lookup Table1/1 -> Divide/3
  Fz/1 -> 1-D Lookup Table1/1, Divide/4, 1-D Lookup Table2/1, 1-D Lookup Table3/1, Divide1/4, 1-D Lookup Table/1
  Divide1/1 -> Square1/1  "s_bar"
  1-D Lookup Table2/1 -> Divide1/2
  1-D Lookup Table3/1 -> Divide1/3
  Switch/1 -> Divide1/1
  Switch1/1 -> Divide/1
  Compute SL Fake/1(SL_fake) -> Switch/3
  Compute SL/1(Out1) -> Switch/1
  Compute SA/1(Out1) -> Switch1/1, Compute SL/1(In1)
  vel/1 -> Compute SL/3(Vg), Selector/1, Compute SL Fake/2(Vg), Selector1/1, Compute SA/3(Vg)
  ang_vel/1 -> Compute SA/2(ang_vel)
  omega/1 -> Compute SL Fake/1(omega), Compute SL/2(omega)
  Steering Model/1(steering) -> Compute SA/1(steering)
  Constant1/1 -> Switch1/3
  Sqrt/1 -> Switch2/1
  Constant2/1 -> Switch2/2
  Selector/1 -> Switch/2
  Selector1/1 -> Switch1/2
  Square/1 -> Sum/1
  Square1/1 -> Sum/2
  CCSA/1 -> Steering Model/1(steering_angle)

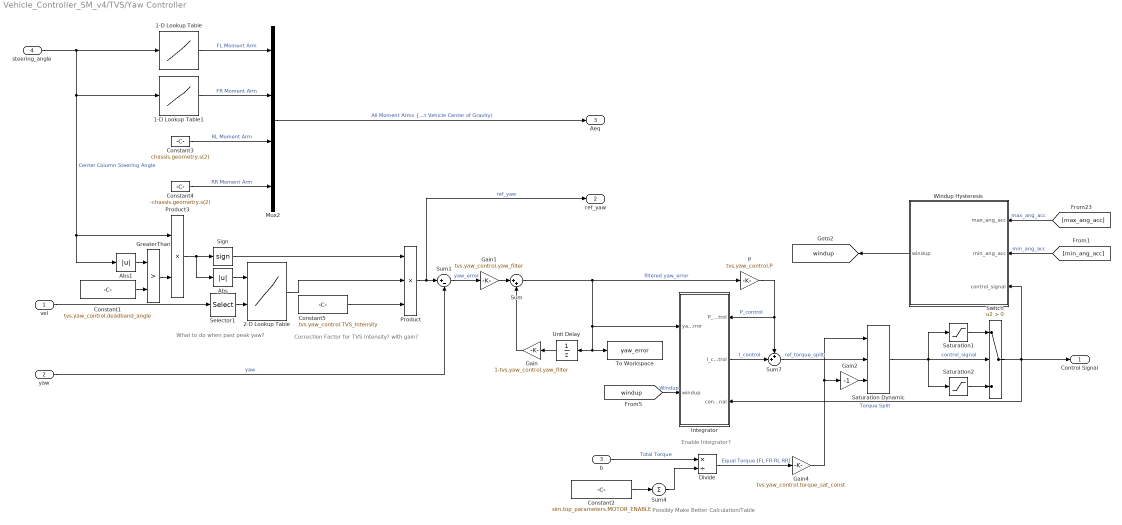
== system Vehicle_Controller_SM_v4/TVS/Yaw Controller ==
  note: Correction Factor for TVS Intensity? with gain?
  note: Enable Integrator?
  note: What to do when past peak yaw?
  note: Possibly Make Better Calculation/Table
  vel : Inport
  yaw : Inport  Port=2  OutDataTypeStr=double  LockScale=on
  b : Inport  Port=3
  steering_angle : Inport  Port=4
  1-D Lookup Table : Lookup_n-D  NumberOfTableDimensions=1  BreakpointsForDimension1=suspension.steering.theta_sweep  Table=suspension.steering.Aeq_left  ExtrapMethod=Clip  InternalRulePriority=Speed  RndMeth=Simplest
  1-D Lookup Table1 : Lookup_n-D  NumberOfTableDimensions=1  BreakpointsForDimension1=suspension.steering.theta_sweep  Table=suspension.steering.Aeq_right  ExtrapMethod=Clip  InternalRulePriority=Speed  RndMeth=Simplest
  2-D Lookup Table : Lookup_n-D  BreakpointsForDimension1=tvs.yaw_control.max_s_bp  BreakpointsForDimension2=tvs.yaw_control.max_v_bp  Table=tvs.yaw_control.max_yaw_table_ref  ExtrapMethod=Clip  InternalRulePriority=Speed  RndMeth=Simplest
      settings: InputPortMap=u0,u1
  Abs : Abs  SaturateOnIntegerOverflow=off
  Abs1 : Abs  SaturateOnIntegerOverflow=off
  Constant1 : Constant  Value=tvs.yaw_control.deadband_angle
  Constant2 : Constant  Value=sim.top_parameters.MOTOR_ENABLE
  Constant3 : Constant  Value=chassis.geometry.s(2)  OutDataTypeStr=Inherit: Inherit via back propagation
  Constant4 : Constant  Value=-chassis.geometry.s(2)  OutDataTypeStr=Inherit: Inherit via back propagation
  Constant5 : Constant  Value=tvs.yaw_control.TVS_Intensity
  Divide : Product  Inputs=*/
  Gain : Gain  Gain=1-tvs.yaw_control.yaw_filter
  Gain1 : Gain  Gain=tvs.yaw_control.yaw_filter
  Gain2 : Gain  Gain=-1
  Gain4 : Gain  Gain=tvs.yaw_control.torque_sat_const
  GreaterThan : RelationalOperator  Operator=>  OutDataTypeStr=boolean  RndMeth=Simplest  InputSameDT=off
  Integrator : Subsystem
      settings: PortSchema="{\"entries\":[{\"content\":{\"sides\":[{\"content\":{\"connectorIds\":[\"In1\",\"In2\"]},\"type\":\"ConnectorPlacement.EquallySpacedRectSide\",\"uuid\":\"8eceed30-5463-482b-9ad9-1d0859eec1e0\"},{\"content\":{\"connectorIds\":[\"In3\",\"Out1\",\"In4\"],\"side\":\"RIGHT\"},\"type\":\"ConnectorPlacement.EquallySpacedRectSide\",\"uuid\":\"ca18b8b2-b2b4-4da4-8362-ca68ae703b33\"},{\"content\":{\"connectorIds\":[],\"side\":\"TOP\"},\"type\":\"ConnectorPlacement.EquallySpacedRectSide\",\"uuid\":\"14e81d29-e47e-408e-961b-b14eadc3d40e\"}]},\"type\":\"ConnectorPlacement.EquallySpacedConnector\",\"uuid\":\"147d3fcd-d0df-4d8b-910b-d1c7e2c77e1f\"}],\"packageUris\":[\"http://schema.mathworks.com/mf0/Connector/R2020b\"],\"version\":\"1.0\"}"
  Mux2 : Mux
  P : Gain  Gain=tvs.yaw_control.P  ParamDataTypeStr=double  OutDataTypeStr=double
  Product : Product  Inputs=3  OutDataTypeStr=Inherit: Inherit via back propagation
  Product3 : Product
  Saturation Dynamic : simulink/Discontinuities/Saturation Dynamic  OutMin=[]  OutMax=[]  OutDataTypeStr=Inherit: Same as second input  OutDataType=fixdt(1, 16)  OutScaling=2^-10  DoSatur=off
  Saturation1 : Saturate  UpperLimit=inf  LowerLimit=tvs.yaw_control.dB
  Saturation2 : Saturate  UpperLimit=-tvs.yaw_control.dB  LowerLimit=-inf
  Selector1 : Selector  InputPortWidth=4  IndexOptions=Index vector (dialog)  Indices=4  OutputSizes=1
  Sign : Signum
  Sum : Sum  Inputs=|++
  Sum1 : Sum  Inputs=|+-  OutDataTypeStr=Inherit: Inherit via back propagation
  Sum4 : Sum  Inputs=+
  Sum7 : Sum  Inputs=++|  OutDataTypeStr=double  SaturateOnIntegerOverflow=on
  Switch : Switch  Criteria=u2 > Threshold  SaturateOnIntegerOverflow=off  InputSameDT=off
  To Workspace : ToWorkspace  VariableName=yaw_error  SaveFormat=Timeseries  SampleTime=-1
  Unit Delay : UnitDelay  SampleTime=-1  HasFrameUpgradeWarning=on
  Windup Hysteresis : Subsystem
  Control Signal : Outport  OutDataTypeStr=double  PortDimensions=1  LockScale=on
  ref_yaw : Outport  Port=2
  Aeq : Outport  Port=3  OutDataTypeStr=double  LockScale=on
  tag scope: windup=global
  wires:
  P/1 -> Sum7/1, Integrator/3(P_control)  "P_control"
  yaw/1 -> Sum1/2  "yaw"
  Integrator/1(I_control) -> Sum7/2  "I_control"
  Sum7/1 -> Saturation Dynamic/2  "ref_torque_split"
  Saturation Dynamic/1 -> Saturation2/1, Saturation1/1, Switch/2  "control_signal"
  Windup Hysteresis/1(windup) -> [windup]
  Sum/1 -> P/1, Unit Delay/1, To Workspace/1, Integrator/1(yaw_error)  "filtered yaw_error"
  [windup] -> Integrator/2(windup)  "Windup"
  Unit Delay/1 -> Gain/1
  Gain/1 -> Sum/2
  Gain1/1 -> Sum/1
  Sum1/1 -> Gain1/1  "yaw_error"
  Switch/1 -> Windup Hysteresis/3(control_signal), Control Signal/1, Integrator/4(control_signal)  "Torque Split"
  Saturation1/1 -> Switch/1
  Saturation2/1 -> Switch/3
  Constant4/1 -> Mux2/4  "RR Moment Arm"
  b/1 -> Divide/1  "Total Torque"
  Constant3/1 -> Mux2/3  "RL Moment Arm"
  1-D Lookup Table/1 -> Mux2/1  "FL Moment Arm"
  1-D Lookup Table1/1 -> Mux2/2  "FR Moment Arm"
  Mux2/1 -> Aeq/1  "All Moment Arms {FL FR RL RR] (about Vehicle Center of Gravity)"
  Divide/1 -> Gain4/1  "Equal Torque [FL FR RL RR]"
  Product/1 -> ref_yaw/1, Sum1/1  "ref_yaw"
  Constant1/1 -> GreaterThan/2
  steering_angle/1 -> 1-D Lookup Table1/1, Product3/1, Abs1/1, 1-D Lookup Table/1  "Center Column Steering Angle"
  vel/1 -> Selector1/1
  Abs/1 -> 2-D Lookup Table/1
  Product3/1 -> Abs/1, Sign/1
  Sign/1 -> Product/1
  Abs1/1 -> GreaterThan/1
  GreaterThan/1 -> Product3/2
  Selector1/1 -> 2-D Lookup Table/2
  [min_ang_acc] -> Windup Hysteresis/2(min_ang_acc)  "min_ang_acc"
  [max_ang_acc] -> Windup Hysteresis/1(max_ang_acc)  "max_ang_acc"
  Gain2/1 -> Saturation Dynamic/3
  Gain4/1 -> Gain2/1, Saturation Dynamic/1
  2-D Lookup Table/1 -> Product/2
  Constant5/1 -> Product/3
  Constant2/1 -> Sum4/1
  Sum4/1 -> Divide/2

== system Vehicle_Controller_SM_v4/TVS/Traction Controller/Compute SA ==
  steering : Inport
  ang_vel : Inport  Port=2
  Vg : Inport  Port=3
  Out1 : Outport

== system Vehicle_Controller_SM_v4/TVS/Traction Controller/Compute SL ==
  In1 : Inport
  omega : Inport  Port=2
  Vg : Inport  Port=3
  Out1 : Outport

== system Vehicle_Controller_SM_v4/TVS/Traction Controller/Compute SL Fake ==
  omega : Inport
  Vg : Inport  Port=2
  Divide : Product  Inputs=*/
  Gain : Gain  Gain=suspension.tire.RE
  Subtract : Sum  Inputs=+-
  SL_fake : Outport
  wires:
  omega/1 -> Gain/1
  Gain/1 -> Subtract/1
  Divide/1 -> SL_fake/1
  Subtract/1 -> Divide/1

== system Vehicle_Controller_SM_v4/TVS/Traction Controller/Steering Model ==
  steering_angle : Inport  OutMin=-130  OutMax=130  OutDataTypeStr=double  LockScale=on
  1-D Lookup Table : Lookup_n-D  NumberOfTableDimensions=1  BreakpointsForDimension1=suspension.steering.theta_sweep  Table=suspension.steering.theta_left  InterpMethod=Cubic spline  InternalRulePriority=Speed  RndMeth=Simplest
  1-D Lookup Table1 : Lookup_n-D  NumberOfTableDimensions=1  BreakpointsForDimension1=suspension.steering.theta_sweep  Table=suspension.steering.theta_right  InterpMethod=Cubic spline  InternalRulePriority=Speed  RndMeth=Simplest
  Bus Creator : BusCreator  Inputs=2
  Mean : dspstat3/Mean  run=off  InputProcessing=Columns as channels (frame based)  reset_popup=None  directionMode=Each column  dimension=1  roiEnable=off  roiType=Rectangles  roiPortion=Entire ROI  roiOutput=Individual statistics for each ROI  roiFlag=off  roundingMode=Floor  overflowMode=off  outputDataTypeStr=Inherit: Same as accumulator  outputMin=[]  outputMax=[]  outputLastDataTypeStr=Inherit: Same as accumulator
  Mux : Mux  Inputs=2
  steering : Outport  OutDataTypeStr=double  LockScale=on
  wires:
  1-D Lookup Table/1 -> Mux/1
  Mean/1 -> Bus Creator/1  "avg_steering_angles"
  Mux/1 -> Bus Creator/2, Mean/1  "steering_angles"
  1-D Lookup Table1/1 -> Mux/2
  Bus Creator/1 -> steering/1
  steering_angle/1 -> 1-D Lookup Table1/1, 1-D Lookup Table/1

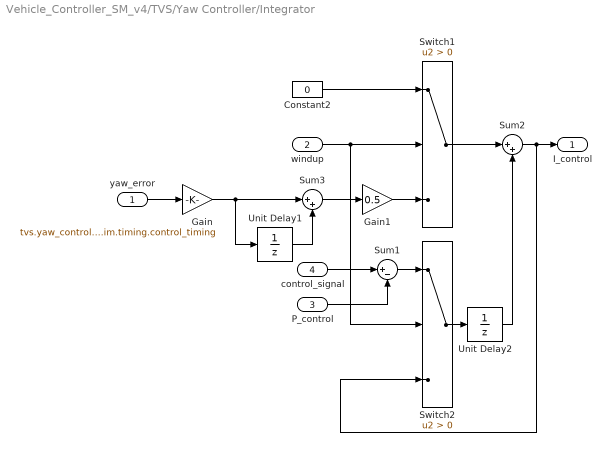
== system Vehicle_Controller_SM_v4/TVS/Yaw Controller/Integrator ==
  yaw_error : Inport
  windup : Inport  Port=2
  P_control : Inport  Port=3
  control_signal : Inport  Port=4
  Constant2 : Constant  Value=0
  Gain : Gain  Gain=tvs.yaw_control.I*sim.timing.control_timing
  Gain1 : Gain  Gain=0.5
  Sum1 : Sum  Inputs=|+-
  Sum2 : Sum  Inputs=|++
  Sum3 : Sum  Inputs=|++
  Switch1 : Switch  Criteria=u2 > Threshold  SaturateOnIntegerOverflow=off  InputSameDT=off
  Switch2 : Switch  Criteria=u2 > Threshold  SaturateOnIntegerOverflow=off  InputSameDT=off
  Unit Delay1 : UnitDelay  SampleTime=-1  HasFrameUpgradeWarning=on
  Unit Delay2 : UnitDelay  SampleTime=-1  HasFrameUpgradeWarning=on
  I_control : Outport
  wires:
  Constant2/1 -> Switch1/1
  windup/1 -> Switch1/2, Switch2/2
  Gain/1 -> Unit Delay1/1, Sum3/1
  Switch1/1 -> Sum2/1
  Gain1/1 -> Switch1/3
  Sum2/1 -> Switch2/3, I_control/1
  Unit Delay1/1 -> Sum3/2
  Sum3/1 -> Gain1/1
  yaw_error/1 -> Gain/1
  control_signal/1 -> Sum1/1
  P_control/1 -> Sum1/2
  Sum1/1 -> Switch2/1
  Switch2/1 -> Unit Delay2/1
  Unit Delay2/1 -> Sum2/2

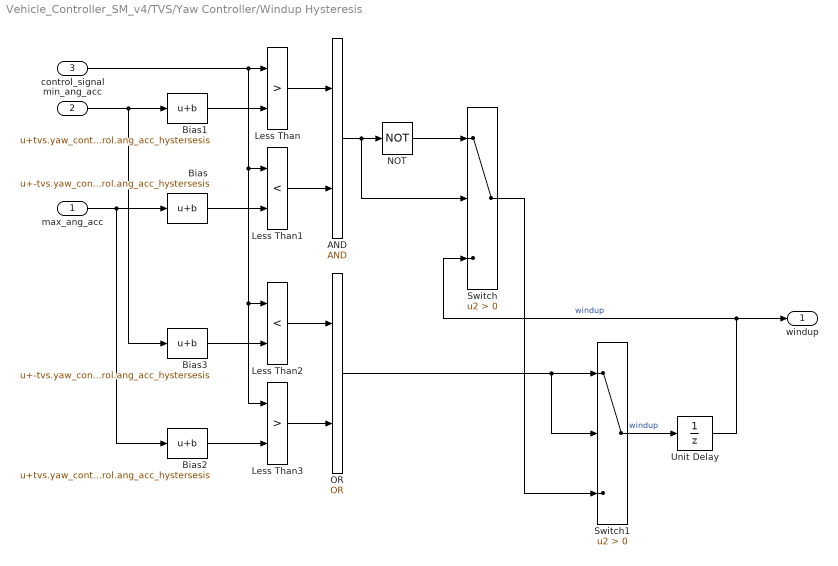
== system Vehicle_Controller_SM_v4/TVS/Yaw Controller/Windup Hysteresis ==
  max_ang_acc : Inport
  min_ang_acc : Inport  Port=2
  control_signal : Inport  Port=3
  AND : Logic  IconShape=distinctive  AllPortsSameDT=off  OutDataTypeStr=boolean
  Bias : Bias  Bias=-tvs.yaw_control.ang_acc_hystersesis  SaturateOnIntegerOverflow=off
  Bias1 : Bias  Bias=tvs.yaw_control.ang_acc_hystersesis  SaturateOnIntegerOverflow=off
  Bias2 : Bias  Bias=tvs.yaw_control.ang_acc_hystersesis  SaturateOnIntegerOverflow=off
  Bias3 : Bias  Bias=-tvs.yaw_control.ang_acc_hystersesis  SaturateOnIntegerOverflow=off
  Less Than : RelationalOperator  Operator=>  OutDataTypeStr=boolean  RndMeth=Simplest  InputSameDT=off
  Less Than1 : RelationalOperator  Operator=<  OutDataTypeStr=boolean  RndMeth=Simplest  InputSameDT=off
  Less Than2 : RelationalOperator  Operator=<  OutDataTypeStr=boolean  RndMeth=Simplest  InputSameDT=off
  Less Than3 : RelationalOperator  Operator=>  OutDataTypeStr=boolean  RndMeth=Simplest  InputSameDT=off
  NOT : Logic  Operator=NOT  IconShape=distinctive  AllPortsSameDT=off  OutDataTypeStr=boolean
  OR : Logic  Operator=OR  IconShape=distinctive  AllPortsSameDT=off  OutDataTypeStr=boolean
  Switch : Switch  Criteria=u2 > Threshold  SaturateOnIntegerOverflow=off  InputSameDT=off
  Switch1 : Switch  Criteria=u2 > Threshold  SaturateOnIntegerOverflow=off  InputSameDT=off
  Unit Delay : UnitDelay  SampleTime=-1  HasFrameUpgradeWarning=on
  windup : Outport
  wires:
  min_ang_acc/1 -> Bias1/1, Bias3/1
  max_ang_acc/1 -> Bias/1, Bias2/1
  Less Than/1 -> AND/1
  Less Than1/1 -> AND/2
  Bias/1 -> Less Than1/2
  Bias1/1 -> Less Than/2
  AND/1 -> Switch/2, NOT/1
  Unit Delay/1 -> Switch/3, windup/1  "windup"
  Bias3/1 -> Less Than2/2
  Bias2/1 -> Less Than3/2
  OR/1 -> Switch1/2, Switch1/1
  Less Than3/1 -> OR/2
  Less Than2/1 -> OR/1
  control_signal/1 -> Less Than2/1, Less Than3/1, Less Than1/1, Less Than/1
  NOT/1 -> Switch/1
  Switch/1 -> Switch1/3
  Switch1/1 -> Unit Delay/1  "windup"

== stateflow chart Vehicle_Controller_SM_v4/State Machine/Mode Selection ==
  note: Aggressive Steering: monitoring rapid increase or decrease in Θ over a short duration signifies aggressive steering input.
      | High Speeds with Steering: first, check the Chassis Absolute Velocity (V_NED) to confirm high speeds, and second, monitor any non-trivial steering input via Θ.
  state ETtoTVSIntent
    en:
    st = [0.5;0;0.5];
  state TVS
    en:
    st = [0;0;1];
  state Equal_Torque
    en:
    st = [1;0;0];
  state DetectDecelerationIntent
    en:
    st = [0.5;0.5;0];
  state DetectHighSpeedDecelerationIntent
    en:
    st = [0;0.5;0.5];
  state Regn
    st = [0;1;0;];
  (default) -> Equal_Torque
  ETtoTVSIntent -> TVS [order 1] : [rateSteer > 100]
  ETtoTVSIntent -> TVS [order 2] : [(V_NED > 30) & (rateSteer > 10)]
  Equal_Torque -> ETtoTVSIntent [order 1] : [(rateSteer > 10)]
  Regn -> TVS [order 1] : [((V_NED > 30) || (rateSteer > 100)) & (Throttle > 0.2)]
  TVS -> ETtoTVSIntent [order 2] : [(rateSteer < 10)]
  ETtoTVSIntent -> Equal_Torque [order 3] : [after(2,second)]
  TVS -> DetectHighSpeedDecelerationIntent [order 1] : [(Throttle < 0.01) && (V_NED >40)]
  DetectHighSpeedDecelerationIntent -> TVS [order 2] : [(slip > 0.2) ]
  Equal_Torque -> DetectDecelerationIntent [order 2] : [Throttle < 0.02]
  Regn -> Equal_Torque [order 2] : [ (Throttle > 0.2)]
  DetectDecelerationIntent -> (junction 40) : [(rateV_NED > 10) || (Brake > 0.1) ]
  (junction 40) -> DetectDecelerationIntent [order 2] : [Throttle > 0.2]
  DetectHighSpeedDecelerationIntent -> Regn [order 1] : [after(1,second)]
  (junction 40) -> Regn [order 1] : [after(1,second)]
  data: st output double size=[3 1]; rateThrottle input double size=[1 1]; Throttle input double size=[1 1]; rateSteer input double size=[1 1]; Steer input double size=[1 1]; Brake input double size=[1 1]; V_NED input double size=[1 1]; rateV_NED input double size=[1 1]; slip input double

== matlab function Vehicle_Controller_SM_v4/Throttle Map/Mode_K_select ==
  data: Mode input; k_OUT output; k_TV input
function k_OUT = fcn(Mode, k_TV)
    if Mode(1) == 1
        k_OUT = k_TV(1,:);
    elseif Mode(2) == 1
        k_OUT = k_TV(2,:);
    else
        k_OUT = k_TV(3,:);
    end
end

== matlab function Vehicle_Controller_SM_v4/Sensor Fusion/NED2VNED ==
  data: rot_map input; state input; ang output; angvel output; pos output; vel output; accel output; mag output; accel_bias output; gyro_bias output; mag_bias output
function [ang,angvel,pos,vel,accel,mag,accel_bias,gyro_bias,mag_bias] = NED2VNED(rot_map, state)
%% Vehicle POSE
ang = state(1:4);                    % quaternion (VNED2SNED)
angvel = state(5:7);                 % chassis angular velocity (rad/s)(VNED)
pos = state(8:10);                   % chassis position (m)(NED)
vel = rot_map*state(11:13);          % chassis velocity (m/s)(VNED)
accel = rot_map*state(14:16);        % chassis acceleration (m/s^2)(VNED)
mag = state(23:25);                  % magnetic field (uT)(NED)

%% Sensor Parameters
accel_bias = rot_map*state(17:19);   % accelerometer bias (m/s^2)(VNED)
gyro_bias = rot_map*state(20:22);    % gyroscope bias (rad/s)(VNED)
mag_bias = state(26:28);             % magnetometer bias (uT)(NED)

end

== matlab function Vehicle_Controller_SM_v4/Sensor Fusion/SNED to VNED ==
  data: accel_VNED output size=[3 1]; gyro_VNED output size=[3 1]; accel_SNED input; gyro_SNED input; mag_SNED input; mag_VNED output size=[3 1]; chassis parameter
function [accel_VNED, gyro_VNED, mag_VNED] = SNED2VNED(accel_SNED, gyro_SNED, mag_SNED, chassis)
%% Define Rotation
IMUNED2VNED = rotmat(quaternion([0 (chassis.geometry.phi - 180) 0],"eulerd","XYZ","frame"),"frame");
MAGNED2VNED = rotmat(quaternion([180 (180 - chassis.geometry.phi) 0],"eulerd","XYZ","frame"),"frame");

%% Coordinate Transformation
accel_VNED = IMUNED2VNED*accel_SNED;  % chassis acceleration (m/s^2)(NED)
gyro_VNED = IMUNED2VNED*gyro_SNED;    % chassis angular velocity (rad/s)(VNED)
mag_VNED = MAGNED2VNED*mag_SNED;      % magnetic field (uT)(NED)

end

== matlab function Vehicle_Controller_SM_v4/Sensor Fusion/fusion ==
  data: count input; count output; rot_map output; velocity input size=[1,3]; state_out output; position input size=[1,3]; acceleration input size=[1,3]; angularVelocity input size=[1,3]; magField input size=[1,3]; state_in input; cov_in input; sim parameter; sensor parameter; cov_out output
function [count, rot_map, state_out, cov_out] = fusion(count, velocity, position ,acceleration,angularVelocity, magField, state_in, cov_in, sim, sensor) 
%% Create Filter
filter = insfilterAsync();
filter.ReferenceLocation = sim.IC.location_lla_IC;
filter.State = state_in;
filter.StateCovariance = cov_in;

filter.QuaternionNoise = sensor.noise.noise_state(1:4);
filter.AngularVelocityNoise = sensor.noise.noise_state(5:7);
filter.PositionNoise = sensor.noise.noise_state(8:10);
filter.VelocityNoise = sensor.noise.noise_state(11:13);
filter.AccelerationNoise = sensor.noise.noise_state(14:16);
filter.GyroscopeBiasNoise = sensor.noise.noise_state(17:19);
filter.AccelerometerBiasNoise = sensor.noise.noise_state(20:22);
filter.GeomagneticVectorNoise = sensor.noise.noise_state(23:25);
filter.MagnetometerBiasNoise = sensor.noise.noise_state(26:28);

%% Sensor Fusion
predict(filter, sim.timing.control_timing);

fuseaccel(filter,acceleration,sensor.imu.covA);
fusegyro(filter,angularVelocity,sensor.imu.covG);
fusemag(filter, magField,sensor.imu.covM);

if ~count
    fusegps(filter,position,sensor.gps.covP,velocity,sensor.gps.covV);
end

count = mod(count + 1, sim.timing.gps_ratio);

[~,rot_map,~] = pose(filter, 'rotmat');

%% Save Fusion State & State Covariance
state_out = filter.State;
cov_out = filter.StateCovariance;

end
